simulink model "ADI_artificial"  (R2019b)
settings: Solver=FixedStepAuto  StartTime=0.0  StopTime=10.0  FixedStep=fixedStepSize  RelTol=1e-3
undefined symbols (not defined in the file): ADI_evChangesDuration, ADI_notAlways1Horizon, ADI_outputTorqueBound, ADI_subsystem1_downThreshold1, ADI_subsystem1_downThreshold2, ADI_subsystem1_downThreshold3, ADI_subsystem1_downThreshold4, ADI_subsystem1_evChangesDuration, ADI_subsystem1_gearOption1, ADI_subsystem1_gearOption2, ADI_subsystem1_speedThreshold, ADI_subsystem2_evChangesDuration, ADI_subsystem2_gear1, ADI_subsystem2_gear2, ADI_subsystem2_notAlwaysHorizon, ADI_subsystem2_speedMin, ADI_subsystem3_downThreshold, ADI_subsystem3_gear, ADI_subsystem3_gearSelectionState, ADI_subsystem3_impellerTorque, ADI_subsystem3_RPM, ADI_subsystem3_upThreshold, ADI_subsystem4_downThreshold, ADI_subsystem4_gear, ADI_subsystem4_gearSelectionState, ADI_subsystem4_notAlways1Horizon, ADI_subsystem4_notAlwaysHorizon, ADI_subsystem4_RPM, ADI_subsystem4_throttle, ADI_subsystem4_upThreshold, ADI_subsystem5_evChanges1Duration, ADI_subsystem5_evChangesDuration, ADI_subsystem5_notAlwaysHorizon, ADI_subsystem5_speedThreshold, artificial_ADI_BTL_constant, artificial_ADI_constant, fixedStepSize
libraries: simulink x11
(part 2 of 2)

== system ADI_artificial/subsystem5/evChanges1 ==
  duration : Inport
  sampleTime : Inport  Port=2
  inputSignal : Inport  Port=3
  Constant1 : Constant  Value=0
  Detect Change1 : simulink/Logic and Bit Operations/Detect Change  vinit=0  OutDataTypeStr=boolean
  Relational Operator1 : RelationalOperator  Operator=>  OutDataTypeStr=boolean  RndMeth=Nearest
  Saturation : Saturate  UpperLimit=Inf  LowerLimit=0
  Subtract : Sum  Inputs=-+
  Switch1 : Switch  Criteria=u2 ~= 0
  Unit Delay1 : UnitDelay  SampleTime=-1  HasFrameUpgradeWarning=on
  evChanges : Outport  VectorParamsAs1DForOutWhenUnconnected=off
  wires:
  Detect Change1/1 -> Switch1/2
  duration/1 -> Switch1/1
  Switch1/1 -> Saturation/1
  inputSignal/1 -> Detect Change1/1
  Constant1/1 -> Relational Operator1/2
  Subtract/1 -> Switch1/3
  Saturation/1 -> Relational Operator1/1, Unit Delay1/1
  Unit Delay1/1 -> Subtract/2
  Relational Operator1/1 -> evChanges/1
  sampleTime/1 -> Subtract/1

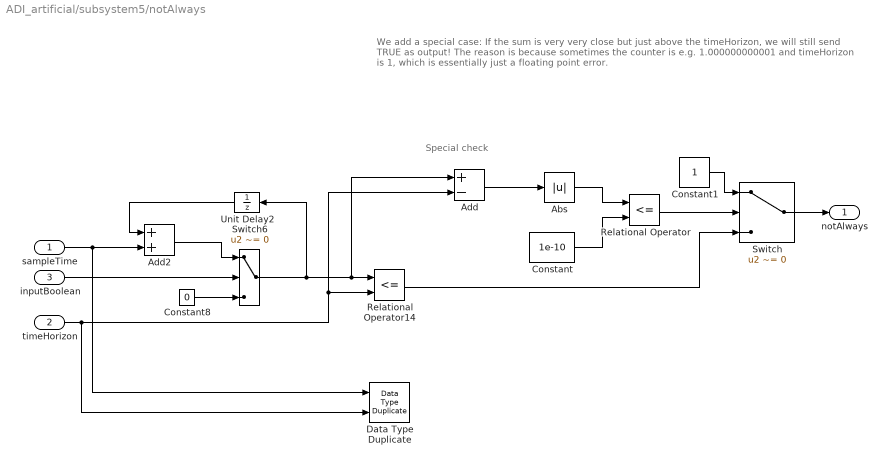
== system ADI_artificial/subsystem5/notAlways ==
  note: Special check
  note: We add a special case:
      | If the sum is very very close but just above the timeHorizon, we will still send TRUE as output!
      |
      | The reason is because sometimes the counter is e.g. 1.000000000001 and timeHorizon is 1, which is essentially just a floating point error.
  sampleTime : Inport
  timeHorizon : Inport  Port=2
  inputBoolean : Inport  Port=3
  Abs : Abs
  Add : Sum  Inputs=+-
  Add2 : Sum
  Constant : Constant  Value=1e-10
  Constant1 : Constant  OutDataTypeStr=boolean
  Constant8 : Constant  Value=0  OutDataTypeStr=Inherit: Inherit via back propagation
  Data Type Duplicate : DataTypeDuplicate
  Relational Operator : RelationalOperator  Operator=<=  OutDataTypeStr=boolean  RndMeth=Simplest
  Relational Operator14 : RelationalOperator  Operator=<=  OutDataTypeStr=boolean  RndMeth=Nearest
  Switch : Switch  Criteria=u2 ~= 0
  Switch6 : Switch  Criteria=u2 ~= 0
  Unit Delay2 : UnitDelay  SampleTime=-1  HasFrameUpgradeWarning=on
  notAlways : Outport  VectorParamsAs1DForOutWhenUnconnected=off
  wires:
  Switch6/1 -> Add/1, Relational Operator14/1, Unit Delay2/1
  timeHorizon/1 -> Add/2, Relational Operator14/2, Data Type Duplicate/2
  Relational Operator14/1 -> Switch/3
  Unit Delay2/1 -> Add2/1
  Add2/1 -> Switch6/1
  sampleTime/1 -> Add2/2, Data Type Duplicate/1
  Constant8/1 -> Switch6/3
  inputBoolean/1 -> Switch6/2
  Add/1 -> Abs/1
  Abs/1 -> Relational Operator/1
  Constant/1 -> Relational Operator/2
  Relational Operator/1 -> Switch/2
  Constant1/1 -> Switch/1
  Switch/1 -> notAlways/1
